simulink model "Sprott_Sliding"  (R2017a)
settings: Solver=VariableStepAuto  StartTime=0.0  StopTime=100  RelTol=1e-3  EnableMultiTasking=on
values from neighbouring files (symbols this model uses):
  c1 = 10    [DataProcessing_Sliding.m]
  c2 = 10    [DataProcessing_Sliding.m]
  c3 = 1    [DataProcessing_Sliding.m]
  W = 0.9    [DataProcessing_Sliding.m]
libraries: dspsnks4 x1, dspvision x1
settings Model: Creator=Luis  LastModifiedBy=Radian
settings DataIOCC: MaxDataPoints=10000000  SaveFormat=Array
settings OptimizationCC: LifeSpan=inf
settings DebuggingCC: MaxConsecutiveZCsMsg=none  SolverPrmCheckMsg=warning  SFUnexpectedBacktrackingDiag=warning  SFNoUnconditionalDefaultTransitionDiag=warning  SFExecutionAtInitializationDiag=none
settings HardwareCC: ProdBitPerPointer=32  ProdBitPerSizeT=32  ProdBitPerPtrDiffT=32  ProdLargestAtomicFloat=None  ProdIntDivRoundTo=Undefined  ProdEndianess=Unspecified  ProdWordSize=32  ProdHWDeviceType=32-bit Generic
settings ModelReferenceCC: PropagateSignalLabelsOutOfModel=off
settings GRTTargetCC: TargetLangStandard=C89/C90 (ANSI)  GeneratePreprocessorConditionals=Disable all
settings ConfigComp: CovMetricSettings=dw  CovHtmlReporting=on  CovSaveCumulativeToWorkspaceVar=on  CovSaveSingleToWorkspaceVar=on  CovExternalEMLEnable=off  CovSFcnEnable=off

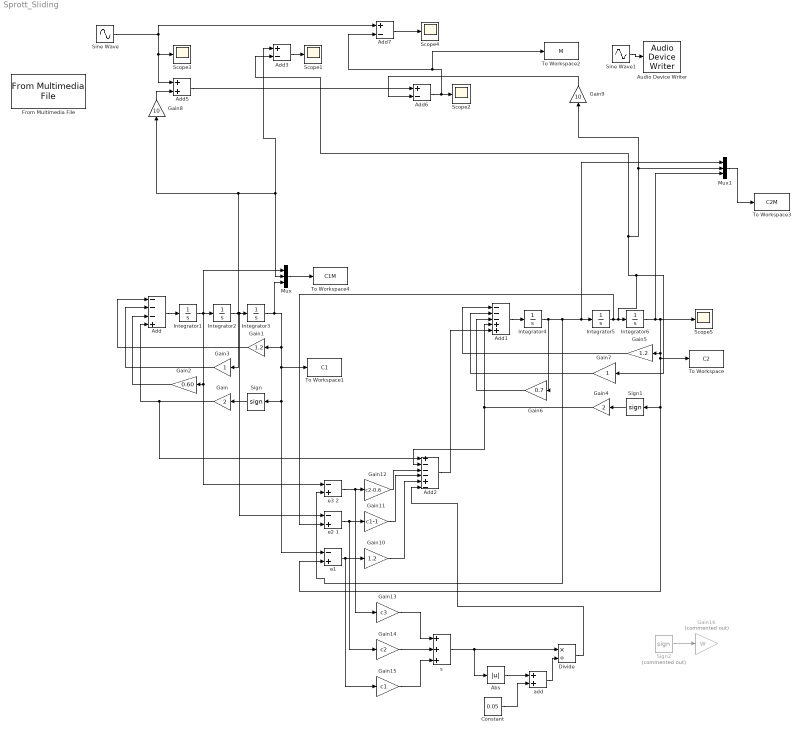
== system Sprott_Sliding ==
  Abs : Abs
  Add : Sum  Inputs=---+
  Add1 : Sum  Inputs=---++
  Add2 : Sum  Inputs=+---+-
  Add3 : Sum  Inputs=+-
  Add5 : Sum
  Add6 : Sum  Inputs=+-
  Add7 : Sum  Inputs=+-
  Audio Device Writer : dspsnks4/Audio Device Writer  Driver=DirectSound  Device=Default  InheritSampleRate=on  SampleRate=44100  BitDepth=16-bit integer  BufferSize=4096  NumBuffers=10  DefaultOutputChannelMapping=on  OutputChannelMapping=1:2  OutputNumUnderrunSamples=off  DriverIdx=1  DeviceWarnFlag=''
  Constant : Constant  Value=0.05
  Divide : Product  Inputs=*/
  From Multimedia File : dspvision/From Multimedia File  inputFilename=speech_dft.mp3  loop=on  numPlays=inf  outputStreams=Audio only  videoDataType=single  audioDataType=double  inheritSampleTime=on  userDefinedSampleTime=1/30  noAudioOutput=off  isIntensityVideo=off  fourcc=RGB  colorVideoFormat=Separate color signals  outputEOF=off  dataOrg=Column-major  audioFrameSize=1  computeAudioFrameSize=off  outSamplingMode=Frame based
      settings: SourceProductBaseCode=VP
  Gain : Gain  Gain=2
  Gain1 : Gain  Gain=1.2
  Gain10 : Gain  Gain=1.2
  Gain11 : Gain  Gain=c1-1
  Gain12 : Gain  Gain=c2-0.6
  Gain13 : Gain  Gain=c3
  Gain14 : Gain  Gain=c2
  Gain15 : Gain  Gain=c1
  Gain16 : Gain  Commented=on  Gain=W
  Gain2 : Gain  Gain=0.60
  Gain3 : Gain
  Gain4 : Gain  Gain=2
  Gain5 : Gain  Gain=1.2
  Gain6 : Gain  Gain=0.7
  Gain7 : Gain
  Gain8 : Gain  Gain=10
  Gain9 : Gain  Gain=10
  Integrator1 : Integrator  InitialCondition=1.1
  Integrator2 : Integrator
  Integrator3 : Integrator  InitialCondition=-1
  Integrator4 : Integrator  InitialCondition=0.1
  Integrator5 : Integrator  InitialCondition=0.1
  Integrator6 : Integrator  InitialCondition=0.1
  Mux : Mux  Inputs=3
  Mux1 : Mux  Inputs=3
  Scope{1..5} (5 alike) : Scope
  Sign : Signum
  Sign1 : Signum
  Sign2 : Signum  Commented=on
  Sine Wave : Sin  Amplitude=.5  Frequency=25  SampleTime=0
  Sine Wave1 : Sin  Amplitude=10  Frequency=2000  SampleTime=2000
  To Workspace : ToWorkspace  VariableName=C2  SaveFormat=Structure With Time  SampleTime=-1
  To Workspace1 : ToWorkspace  VariableName=C1  SaveFormat=Structure With Time  SampleTime=-1
  To Workspace2 : ToWorkspace  VariableName=M  SaveFormat=Structure With Time  SampleTime=-1
  To Workspace3 : ToWorkspace  VariableName=C2M  SaveFormat=Structure With Time  SampleTime=-1
  To Workspace4 : ToWorkspace  VariableName=C1M  SaveFormat=Structure With Time  SampleTime=-1
  add : Sum
  "e1 " : Sum  Inputs=-+
  e2 1 : Sum  Inputs=-+
  e3 2 : Sum  Inputs=-+
  s : Sum  Inputs=+++
  wires:
  Integrator1/1 -> e3 2/1, Gain2/1, Mux/1, Integrator2/1
  Integrator2/1 -> Mux/2, Add3/1, Gain8/1, Gain3/1, e2 1/1, Integrator3/1
  Sign/1 -> Gain/1
  Gain/1 -> Add2/1, Add/4
  Gain2/1 -> Add/3
  Integrator3/1 -> "e1 "/1, Sign/1, To Workspace1/1, Gain1/1, Mux/3
  Gain1/1 -> Add/1
  Gain3/1 -> Add/2
  Add/1 -> Integrator1/1
  Integrator4/1 -> e3 2/2, Mux1/1, Integrator5/1, Gain6/1
  Integrator5/1 -> e2 1/2, Integrator6/1, Add3/2, Mux1/2, Gain9/1, Gain7/1
  Sign1/1 -> Gain4/1
  Gain4/1 -> Add2/2, Add1/4
  Gain6/1 -> Add1/3
  Integrator6/1 -> Mux1/3, Scope5/1, "e1 "/2, Sign1/1, To Workspace/1, Gain5/1
  Gain5/1 -> Add1/1
  Gain7/1 -> Add1/2
  Add1/1 -> Integrator4/1
  Gain8/1 -> Add5/2
  Add5/1 -> Add6/1
  Gain9/1 -> Add6/2
  Mux/1 -> To Workspace4/1
  Add6/1 -> Add7/2, To Workspace2/1, Scope2/1
  Add3/1 -> Scope1/1
  Sine Wave/1 -> Add5/1, Scope3/1, Add7/1
  Add7/1 -> Scope4/1
  Mux1/1 -> To Workspace3/1
  "e1 "/1 -> Gain10/1, Gain15/1
  e2 1/1 -> Gain11/1, Gain14/1
  e3 2/1 -> Gain13/1, Gain12/1
  Gain10/1 -> Add2/5
  Gain11/1 -> Add2/4
  Gain12/1 -> Add2/3
  Gain13/1 -> s/1
  Gain14/1 -> s/2
  Gain15/1 -> s/3
  Sign2/1 -> Gain16/1
  Add2/1 -> Add1/5
  s/1 -> Abs/1, Divide/1
  Abs/1 -> add/1
  add/1 -> Divide/2
  Constant/1 -> add/2
  Divide/1 -> Add2/6
  Sine Wave1/1 -> Audio Device Writer/1
